simulink model "Feedback_control"  (R2018a)
settings: Solver=VariableStepAuto  StartTime=0.0  StopTime=10.0  RelTol=1e-3
values from neighbouring files (symbols this model uses):
  cf = 0.25    [Part2_Analyse.m]    (also in Part3_Asservissement.m)
  cp = 0.0107    [Part2_Analyse.m]    (also in Part3_Asservissement.m)
  ct = 0.783 * 1e-3    (= 0.000783)    [Part2_Analyse.m]    (also in Part3_Asservissement.m)
  g = 9.81    [Part2_Analyse.m]    (also in Part3_Asservissement.m)
  Ixx = 0.0686 * 1e-3    (= 6.86e-05)    [Part2_Analyse.m]    (also in Part3_Asservissement.m)
  Iyy = 0.092 * 1e-3    (= 9.2e-05)    [Part2_Analyse.m]    (also in Part3_Asservissement.m)
  Izz = 0.1366 * 1e-3    (= 0.0001366)    [Part2_Analyse.m]    (also in Part3_Asservissement.m)
  K_lmi = Y1/W1    [Part3_Asservissement.m]
  m = 0.068    [Part2_Analyse.m]    (also in Part3_Asservissement.m)
  r = 0.0624    [Part2_Analyse.m]    (also in Part3_Asservissement.m)
settings Model: Creator=ridaa  LastModifiedBy=ridaa

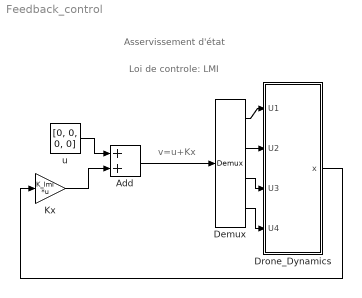
== system Feedback_control ==
  note: Loi de controle: LMI
  note: Asservissement d'état
  note: v=u+Kx
  Add : Sum
  Demux : Demux
  Drone_Dynamics : Subsystem
  Kx : Gain  Gain=K_lmi  Multiplication=Matrix(K*u)
  u : Constant  Value=[0, 0, 0, 0]
  wires:
  Demux/1 -> Drone_Dynamics/1(U1)
  Demux/2 -> Drone_Dynamics/2(U2)
  Demux/3 -> Drone_Dynamics/3(U3)
  Demux/4 -> Drone_Dynamics/4(U4)
  Kx/1 -> Add/2
  Add/1 -> Demux/1
  u/1 -> Add/1
  Drone_Dynamics/1("x ") -> Kx/1

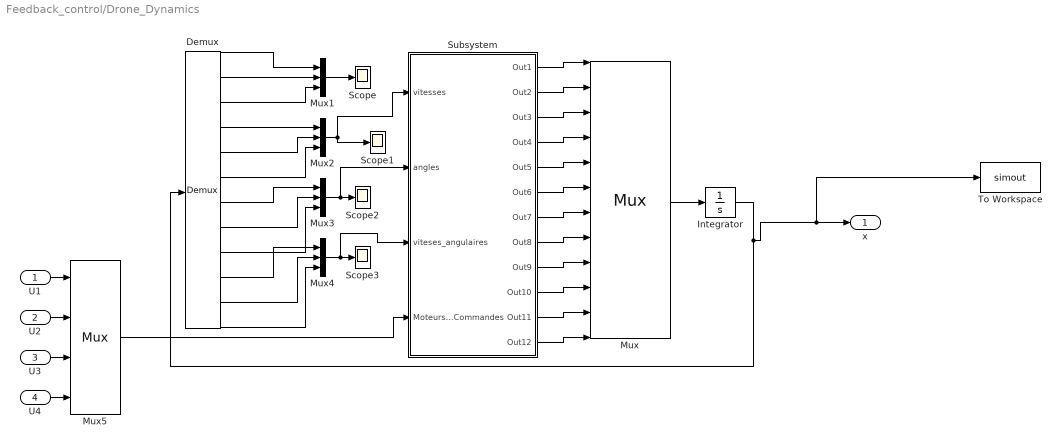
== system Feedback_control/Drone_Dynamics ==
  U1 : Inport
  U2 : Inport  Port=2
  U3 : Inport  Port=3
  U4 : Inport  Port=4
  Demux : Demux  Outputs=12
  Integrator : Integrator  InitialCondition=[0.1,0.1,0.1,0,0,0,0,0,0,0,0,0]
  Mux : Mux  Inputs=12
  Mux{1..4} (4 alike) : Mux  Inputs=3
  Mux5 : Mux
  Scope{,1..3} (4 alike) : Scope
  Subsystem : Subsystem
  To Workspace : ToWorkspace  VariableName=simout  SaveFormat=Structure With Time  SampleTime=-1
  "x " : Outport
  wires:
  Mux2/1 -> Subsystem/1(vitesses), Scope1/1
  Subsystem/5(Out5) -> Mux/5
  Demux/3 -> Mux1/3
  Demux/8 -> Mux3/2
  Integrator/1 -> To Workspace/1, "x "/1, Demux/1
  Subsystem/9(Out9) -> Mux/9
  Mux3/1 -> Subsystem/2(angles), Scope2/1
  Demux/2 -> Mux1/2
  Subsystem/12(Out12) -> Mux/12
  Subsystem/3(Out3) -> Mux/3
  Subsystem/1(Out1) -> Mux/1
  Demux/12 -> Mux4/3
  Subsystem/2(Out2) -> Mux/2
  Subsystem/10(Out10) -> Mux/10
  Demux/11 -> Mux4/2
  Mux4/1 -> Subsystem/3(viteses_angulaires), Scope3/1
  Subsystem/7(Out7) -> Mux/7
  Subsystem/6(Out6) -> Mux/6
  Demux/5 -> Mux2/2
  Mux1/1 -> Scope/1
  Demux/4 -> Mux2/1
  Demux/9 -> Mux3/3
  Mux/1 -> Integrator/1
  Subsystem/8(Out8) -> Mux/8
  Demux/6 -> Mux2/3
  Subsystem/4(Out4) -> Mux/4
  Subsystem/11(Out11) -> Mux/11
  Demux/1 -> Mux1/1
  Mux5/1 -> Subsystem/4(Moteurs Commandes)
  Demux/10 -> Mux4/1
  Demux/7 -> Mux3/1
  U4/1 -> Mux5/4
  U3/1 -> Mux5/3
  U2/1 -> Mux5/2
  U1/1 -> Mux5/1

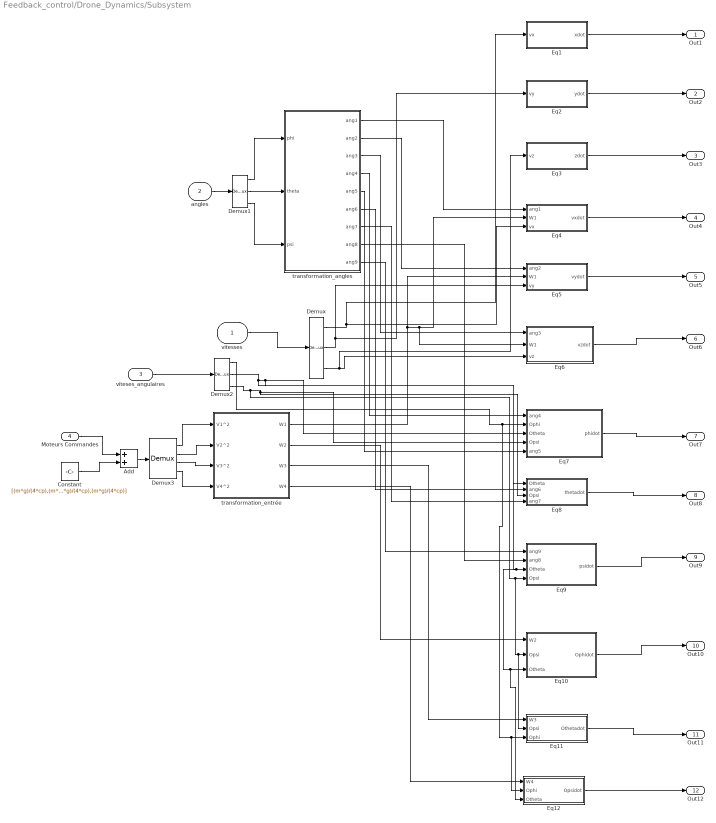
== system Feedback_control/Drone_Dynamics/Subsystem ==
  vitesses : Inport
  angles : Inport  Port=2
  viteses_angulaires : Inport  Port=3
  Moteurs Commandes : Inport  Port=4
  Add : Sum
  Constant : Constant  Value=[(m*g)/(4*cp),(m*g)/(4*cp),(m*g)/(4*cp),(m*g)/(4*cp)]
  Demux : Demux  Outputs=3
  Demux1 : Demux  Outputs=3
  Demux2 : Demux  Outputs=3
  Demux3 : Demux
  Eq1 : Subsystem
  Eq10 : Subsystem
  Eq11 : Subsystem
  Eq12 : Subsystem
  Eq2 : Subsystem
  Eq3 : Subsystem
  Eq4 : Subsystem
  Eq5 : Subsystem
  Eq6 : Subsystem
  Eq7 : Subsystem
  Eq8 : Subsystem
  Eq9 : Subsystem
  transformation_angles : Subsystem
  transformation_entrée : Subsystem
  Out1 : Outport
  Out2 : Outport  Port=2
  Out3 : Outport  Port=3
  Out4 : Outport  Port=4
  Out5 : Outport  Port=5
  Out6 : Outport  Port=6
  Out7 : Outport  Port=7
  Out8 : Outport  Port=8
  Out9 : Outport  Port=9
  Out10 : Outport  Port=10
  Out11 : Outport  Port=11
  Out12 : Outport  Port=12
  wires:
  Eq1/1(xdot) -> Out1/1
  Eq2/1(ydot) -> Out2/1
  Eq3/1(zdot) -> Out3/1
  Eq4/1(vxdot) -> Out4/1
  Eq6/1("vzdot ") -> Out6/1
  Eq5/1("vydot ") -> Out5/1
  Eq7/1("phidot ") -> Out7/1
  Eq9/1("psidot ") -> Out9/1
  Eq8/1(thetadot) -> Out8/1
  Eq10/1(Ophidot) -> Out10/1
  Eq11/1(Othetadot) -> Out11/1
  Eq12/1(Opsidot) -> Out12/1
  vitesses/1 -> Demux/1
  angles/1 -> Demux1/1
  viteses_angulaires/1 -> Demux2/1
  Demux1/1 -> transformation_angles/1(phi)
  Demux1/2 -> transformation_angles/2("theta ")
  Demux1/3 -> transformation_angles/3("psi ")
  transformation_angles/1(ang1) -> Eq4/1(ang1)
  transformation_angles/2(ang2) -> Eq5/1(ang2)
  transformation_angles/3(ang3) -> Eq6/1(ang3)
  transformation_angles/4(ang4) -> Eq7/1("ang4 ")
  transformation_angles/5(ang5) -> Eq7/5(ang5)
  transformation_angles/6(ang6) -> Eq8/2(ang6)
  transformation_angles/7(ang7) -> Eq8/4(ang7)
  transformation_angles/8(ang8) -> Eq9/2(ang8)
  transformation_angles/9(ang9) -> Eq9/1("ang9 ")
  transformation_entrée/1(W1) -> Eq5/2(W1), Eq6/2(W1), Eq4/2(W1)
  transformation_entrée/2(W2) -> Eq10/1(W2)
  transformation_entrée/3("W3 ") -> Eq11/1(W3)
  transformation_entrée/4(W4) -> Eq12/1(W4)
  Demux/1 -> Eq1/1(vx), Eq4/3(vx)
  Demux/2 -> Eq2/1(vy), Eq5/3(vy)
  Demux/3 -> Eq3/1(vz), Eq6/3(vz)
  Demux2/1 -> Eq12/2(Ophi), Eq11/3(Ophi), Eq7/2(Ophi)
  Demux2/2 -> Eq8/1(Otheta), Eq12/3(Otheta), Eq10/3(Otheta), Eq9/3(Otheta), Eq7/3(Otheta)
  Demux2/3 -> Eq11/2(Opsi), Eq10/2(Opsi), Eq9/4(Opsi), Eq8/3(Opsi), Eq7/4(Opsi)
  Demux3/1 -> transformation_entrée/1(V1^2)
  Demux3/2 -> transformation_entrée/2(V2^2)
  Demux3/3 -> transformation_entrée/3(V3^2)
  Demux3/4 -> transformation_entrée/4(V4^2)
  Moteurs Commandes/1 -> Add/1
  Constant/1 -> Add/2
  Add/1 -> Demux3/1

== system Feedback_control/Drone_Dynamics/Subsystem/Eq1 ==
  vx : Inport
  xdot : Outport
  wires:
  vx/1 -> xdot/1

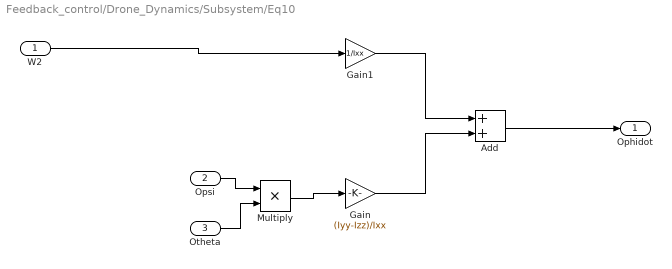
== system Feedback_control/Drone_Dynamics/Subsystem/Eq10 ==
  W2 : Inport
  Opsi : Inport  Port=2
  Otheta : Inport  Port=3
  Add : Sum
  Gain : Gain  Gain=(Iyy-Izz)/Ixx
  Gain1 : Gain  Gain=1/Ixx
  Multiply : Product
  Ophidot : Outport
  wires:
  W2/1 -> Gain1/1
  Opsi/1 -> Multiply/1
  Otheta/1 -> Multiply/2
  Multiply/1 -> Gain/1
  Gain1/1 -> Add/1
  Gain/1 -> Add/2
  Add/1 -> Ophidot/1

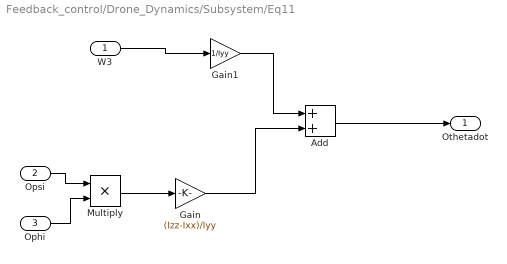
== system Feedback_control/Drone_Dynamics/Subsystem/Eq11 ==
  W3 : Inport
  Opsi : Inport  Port=2
  Ophi : Inport  Port=3
  Add : Sum
  Gain : Gain  Gain=(Izz-Ixx)/Iyy
  Gain1 : Gain  Gain=1/Iyy
  Multiply : Product
  Othetadot : Outport
  wires:
  Gain/1 -> Add/2
  Add/1 -> Othetadot/1
  Ophi/1 -> Multiply/2
  Multiply/1 -> Gain/1
  Opsi/1 -> Multiply/1
  Gain1/1 -> Add/1
  W3/1 -> Gain1/1

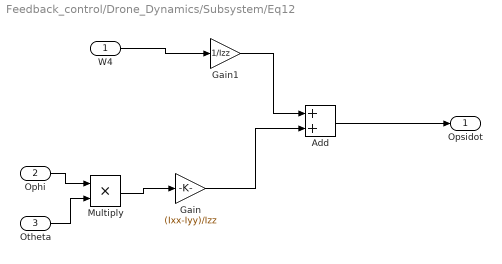
== system Feedback_control/Drone_Dynamics/Subsystem/Eq12 ==
  W4 : Inport
  Ophi : Inport  Port=2
  Otheta : Inport  Port=3
  Add : Sum
  Gain : Gain  Gain=(Ixx-Iyy)/Izz
  Gain1 : Gain  Gain=1/Izz
  Multiply : Product
  Opsidot : Outport
  wires:
  Gain/1 -> Add/2
  Add/1 -> Opsidot/1
  Otheta/1 -> Multiply/2
  Multiply/1 -> Gain/1
  Ophi/1 -> Multiply/1
  Gain1/1 -> Add/1
  W4/1 -> Gain1/1

== system Feedback_control/Drone_Dynamics/Subsystem/Eq2 ==
  vy : Inport
  ydot : Outport
  wires:
  vy/1 -> ydot/1

== system Feedback_control/Drone_Dynamics/Subsystem/Eq3 ==
  vz : Inport
  zdot : Outport
  wires:
  vz/1 -> zdot/1

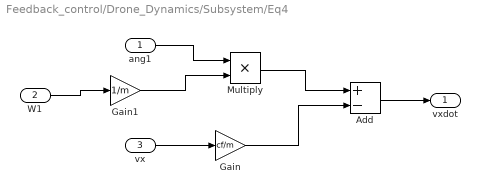
== system Feedback_control/Drone_Dynamics/Subsystem/Eq4 ==
  ang1 : Inport
  W1 : Inport  Port=2
  vx : Inport  Port=3
  Add : Sum  Inputs=+-
  Gain : Gain  Gain=cf/m
  Gain1 : Gain  Gain=1/m
  Multiply : Product
  vxdot : Outport
  wires:
  Add/1 -> vxdot/1
  vx/1 -> Gain/1
  Gain/1 -> Add/2
  ang1/1 -> Multiply/1
  Multiply/1 -> Add/1
  Gain1/1 -> Multiply/2
  W1/1 -> Gain1/1

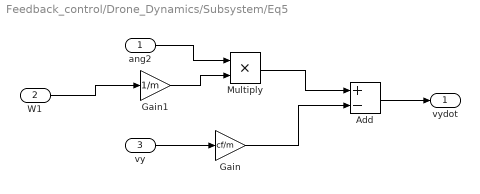
== system Feedback_control/Drone_Dynamics/Subsystem/Eq5 ==
  ang2 : Inport
  W1 : Inport  Port=2
  vy : Inport  Port=3
  Add : Sum  Inputs=+-
  Gain : Gain  Gain=cf/m
  Gain1 : Gain  Gain=1/m
  Multiply : Product
  "vydot " : Outport
  wires:
  vy/1 -> Gain/1
  Add/1 -> "vydot "/1
  ang2/1 -> Multiply/1
  Gain/1 -> Add/2
  Multiply/1 -> Add/1
  Gain1/1 -> Multiply/2
  W1/1 -> Gain1/1

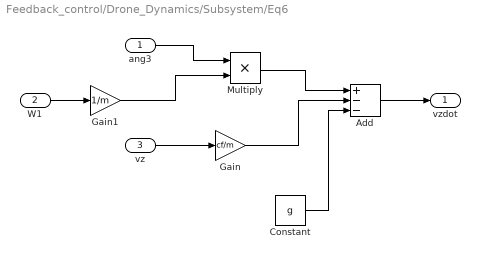
== system Feedback_control/Drone_Dynamics/Subsystem/Eq6 ==
  ang3 : Inport
  W1 : Inport  Port=2
  vz : Inport  Port=3
  Add : Sum  Inputs=+--
  Constant : Constant  Value=g
  Gain : Gain  Gain=cf/m
  Gain1 : Gain  Gain=1/m
  Multiply : Product
  "vzdot " : Outport
  wires:
  Multiply/1 -> Add/1
  Add/1 -> "vzdot "/1
  ang3/1 -> Multiply/1
  Gain/1 -> Add/2
  vz/1 -> Gain/1
  Constant/1 -> Add/3
  Gain1/1 -> Multiply/2
  W1/1 -> Gain1/1

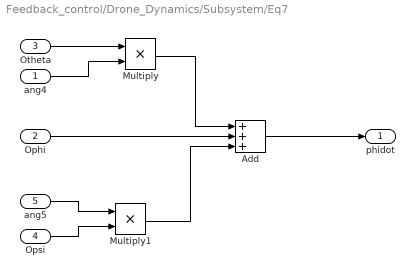
== system Feedback_control/Drone_Dynamics/Subsystem/Eq7 ==
  "ang4 " : Inport
  Ophi : Inport  Port=2
  Otheta : Inport  Port=3
  Opsi : Inport  Port=4
  ang5 : Inport  Port=5
  Add : Sum  Inputs=+++
  Multiply : Product
  Multiply1 : Product
  "phidot " : Outport
  wires:
  Ophi/1 -> Add/2
  Otheta/1 -> Multiply/1
  "ang4 "/1 -> Multiply/2
  Multiply/1 -> Add/1
  ang5/1 -> Multiply1/1
  Opsi/1 -> Multiply1/2
  Multiply1/1 -> Add/3
  Add/1 -> "phidot "/1

== system Feedback_control/Drone_Dynamics/Subsystem/Eq8 ==
  Otheta : Inport
  ang6 : Inport  Port=2
  Opsi : Inport  Port=3
  ang7 : Inport  Port=4
  Add : Sum  Inputs=+-
  Multiply : Product
  Multiply1 : Product
  thetadot : Outport
  wires:
  Otheta/1 -> Multiply/1
  ang6/1 -> Multiply/2
  Opsi/1 -> Multiply1/1
  ang7/1 -> Multiply1/2
  Multiply1/1 -> Add/2
  Multiply/1 -> Add/1
  Add/1 -> thetadot/1

== system Feedback_control/Drone_Dynamics/Subsystem/Eq9 ==
  "ang9 " : Inport
  ang8 : Inport  Port=2
  Otheta : Inport  Port=3
  Opsi : Inport  Port=4
  Add : Sum
  Multiply : Product
  Multiply1 : Product
  "psidot " : Outport
  wires:
  ang8/1 -> Multiply/1
  Otheta/1 -> Multiply/2
  "ang9 "/1 -> Multiply1/1
  Opsi/1 -> Multiply1/2
  Multiply/1 -> Add/1
  Multiply1/1 -> Add/2
  Add/1 -> "psidot "/1

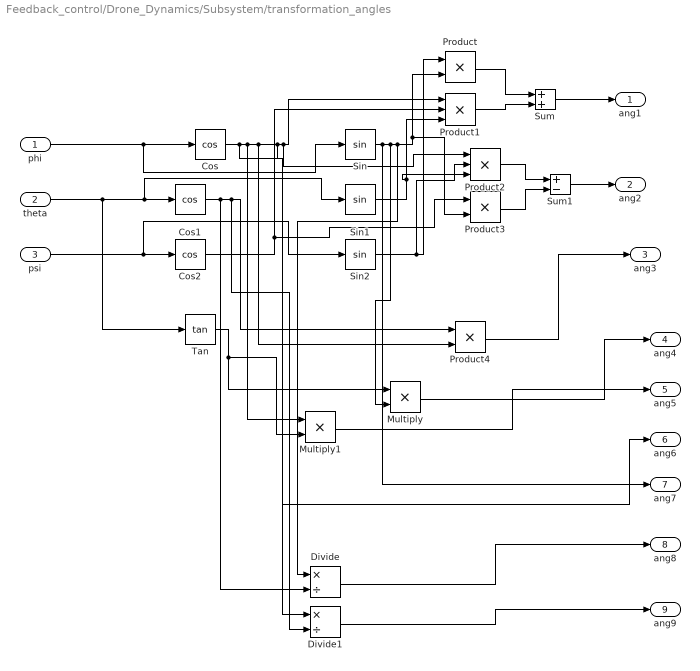
== system Feedback_control/Drone_Dynamics/Subsystem/transformation_angles ==
  phi : Inport
  "theta " : Inport  Port=2
  "psi " : Inport  Port=3
  Cos : Trigonometry  Operator=cos
  Cos1 : Trigonometry  Operator=cos
  Cos2 : Trigonometry  Operator=cos
  Divide : Product  Inputs=*/
  Divide1 : Product  Inputs=*/
  Multiply : Product
  Multiply1 : Product
  Product : Product
  Product1 : Product  Inputs=3
  Product2 : Product  Inputs=3
  Product3 : Product
  Product4 : Product
  Sin : Trigonometry
  Sin1 : Trigonometry
  Sin2 : Trigonometry
  Sum : Sum
  Sum1 : Sum  Inputs=+-
  Tan : Trigonometry  Operator=tan
  ang1 : Outport
  ang2 : Outport  Port=2
  ang3 : Outport  Port=3
  ang4 : Outport  Port=4
  ang5 : Outport  Port=5
  ang6 : Outport  Port=6
  ang7 : Outport  Port=7
  ang8 : Outport  Port=8
  ang9 : Outport  Port=9
  wires:
  "psi "/1 -> Sin2/1, Cos2/1
  phi/1 -> Sin/1, Cos/1
  "theta "/1 -> Tan/1, Sin1/1, Cos1/1
  Sin2/1 -> Product2/2, Product/1
  Sin/1 -> ang7/1, Multiply/2, Divide/1, Product3/2, Product/2
  Cos/1 -> Divide1/1, Multiply1/1, Product4/2, ang6/1, Product2/1, Product1/1
  Cos2/1 -> Product3/1, Product1/2
  Sin1/1 -> Product2/3, Product1/3
  Product/1 -> Sum/1
  Product1/1 -> Sum/2
  Sum/1 -> ang1/1
  Product2/1 -> Sum1/1
  Product3/1 -> Sum1/2
  Sum1/1 -> ang2/1
  Cos1/1 -> Divide/2, Divide1/2, Product4/1
  Product4/1 -> ang3/1
  Tan/1 -> Multiply1/2, Multiply/1
  Multiply/1 -> ang4/1
  Multiply1/1 -> ang5/1
  Divide/1 -> ang8/1
  Divide1/1 -> ang9/1

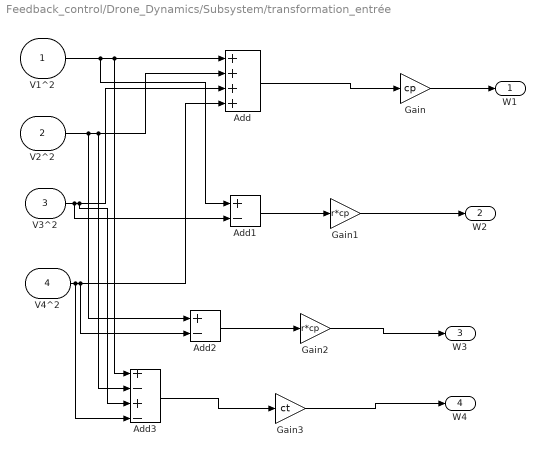
== system Feedback_control/Drone_Dynamics/Subsystem/transformation_entrée ==
  V1^2 : Inport
  V2^2 : Inport  Port=2
  V3^2 : Inport  Port=3
  V4^2 : Inport  Port=4
  Add : Sum  Inputs=++++
  Add1 : Sum  Inputs=+-
  Add2 : Sum  Inputs=+-
  Add3 : Sum  Inputs=+-+-
  Gain : Gain  Gain=cp
  Gain1 : Gain  Gain=r*cp
  Gain2 : Gain  Gain=r*cp
  Gain3 : Gain  Gain=ct
  W1 : Outport
  W2 : Outport  Port=2
  "W3 " : Outport  Port=3
  W4 : Outport  Port=4
  wires:
  V4^2/1 -> Add3/4, Add2/2, Add/4
  V1^2/1 -> Add1/1, Add3/1, Add/1
  V2^2/1 -> Add2/1, Add3/2, Add/2
  V3^2/1 -> Add1/2, Add3/3, Add/3
  Add/1 -> Gain/1
  Gain/1 -> W1/1
  Add1/1 -> Gain1/1
  Gain1/1 -> W2/1
  Gain2/1 -> "W3 "/1
  Add2/1 -> Gain2/1
  Gain3/1 -> W4/1
  Add3/1 -> Gain3/1
